simulink model "window_and_fft_test_v3"  (R2012b)
settings: Solver=ode45  StartTime=0.0  StopTime=100000  RelTol=1e-3
values from neighbouring files (symbols this model uses):
  Fs = 640e6    (= 640000000)    [filter_coefficients.m]    (also in filter_design.m; filter_design_getting_order.m)
undefined symbols (not defined in the file or in its folder): get, pfb_coeff_gen_calc, sided, Two, xlipgetpartsetting
undefined symbols (not defined in the file): A_cos, A_sin, B_cos, B_sin, C_cos, C_sin, casper_coef, D_cos, D_sin
libraries: xbsIndex_r4 x6921, casper_library_misc x45, casper_library_delays x25, dspsnks4 x17, dspspect3 x8, dspsigops x4, xps_library x2, xbsReplacements_r4 x2, casper_library_pfbs x2, simulink x1
(part 2 of 85)

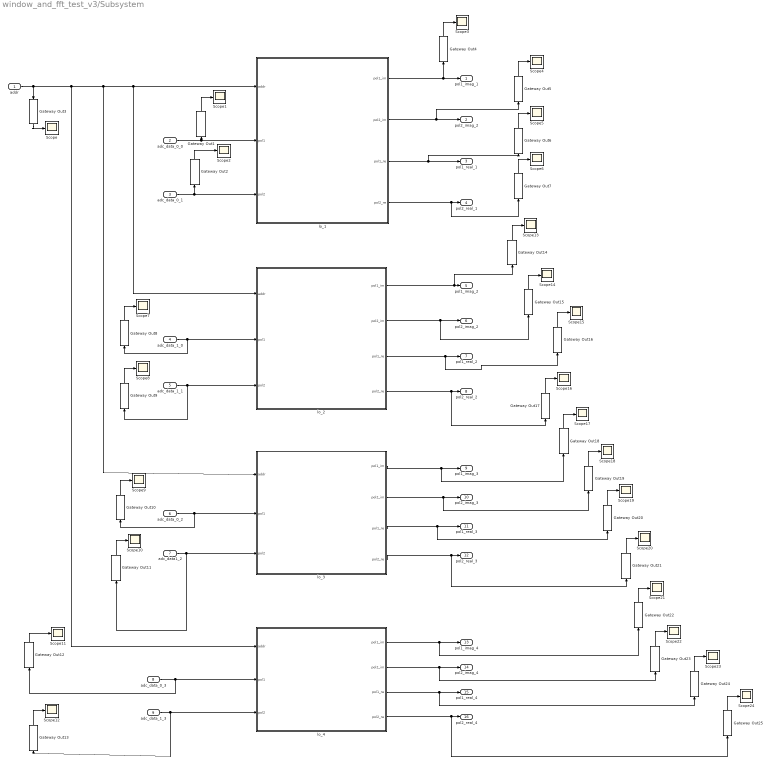
== system window_and_fft_test_v3/Subsystem ==
  addr : Inport
  adc_data_0_0 : Inport  Port=2
  adc_data_0_1 : Inport  Port=3
  adc_data_1_0 : Inport  Port=4
  adc_data_1_1 : Inport  Port=5
  adc_data_0_2 : Inport  Port=6
  adc_data1_2 : Inport  Port=7
  adc_data_0_3 : Inport  Port=8
  adc_data_1_3 : Inport  Port=9
  Gateway Out{1..25} (25 alike) : xbsIndex_r4/Gateway Out  inherit_from_input=on  hdl_port=on  timing_constraint=None  locs_specified=off  LOCs={}  UseAsDAC=off  DACChannel='1'  block_type=gatewayout
  Scope{,1..24} (25 alike) : Scope
      Scope settings: SaveName=ScopeData4
      Scope1 settings: YMin=-0.11  YMax=0.11  SaveName=ScopeData5
      Scope10 settings: YMin=-0.11  YMax=0.11  SaveName=ScopeData19
      Scope11 settings: YMin=-0.11  YMax=0.11  SaveName=ScopeData20
      Scope12 settings: YMin=-0.11  YMax=0.11  SaveName=ScopeData21
      Scope13 settings: YMin=-0.11  YMax=0.11  SaveName=ScopeData22
      Scope14 settings: YMin=-0.11  YMax=0.11  SaveName=ScopeData23
      Scope15 settings: YMin=-0.11  YMax=0.11  SaveName=ScopeData24
      Scope16 settings: YMin=-0.11  YMax=0.11  SaveName=ScopeData25
      Scope17 settings: YMin=-0.11  YMax=0.11  SaveName=ScopeData26
      Scope18 settings: YMin=-0.11  YMax=0.11  SaveName=ScopeData27
      Scope19 settings: YMin=-0.11  YMax=0.11  SaveName=ScopeData28
      Scope2 settings: YMin=-0.11  YMax=0.11  SaveName=ScopeData6
      Scope20 settings: YMin=-0.11  YMax=0.11  SaveName=ScopeData29
      Scope21 settings: YMin=-0.11  YMax=0.11  SaveName=ScopeData30
      Scope22 settings: YMin=-0.11  YMax=0.11  SaveName=ScopeData31
      Scope23 settings: YMin=-0.11  YMax=0.11  SaveName=ScopeData32
      Scope24 settings: YMin=-0.11  YMax=0.11  SaveName=ScopeData33
      Scope3 settings: YMin=-0.11  YMax=0.11  SaveName=ScopeData12
      Scope4 settings: YMin=-0.11  YMax=0.11  SaveName=ScopeData13
      Scope5 settings: YMin=-0.11  YMax=0.11  SaveName=ScopeData14
      Scope6 settings: YMin=-0.11  YMax=0.11  SaveName=ScopeData15
      Scope7 settings: YMin=-0.11  YMax=0.11  SaveName=ScopeData16
      Scope8 settings: YMin=-0.11  YMax=0.11  SaveName=ScopeData17
      Scope9 settings: YMin=-0.11  YMax=0.11  SaveName=ScopeData18
  lo_1 : Subsystem  AncestorBlock=gbt_library/complex_mix_lo
  lo_2 : Subsystem  AncestorBlock=gbt_library/complex_mix_lo
  lo_3 : Subsystem  AncestorBlock=gbt_library/complex_mix_lo
  lo_4 : Subsystem  AncestorBlock=gbt_library/complex_mix_lo
  pol1_imag_1 : Outport
  pol2_imag_2 : Outport  Port=2
  pol1_real_1 : Outport  Port=3
  pol2_real_1 : Outport  Port=4
  pol1_imag_2 : Outport  Port=5
  "pol2_imag_2 " : Outport  Port=6
  pol1_real_2 : Outport  Port=7
  pol2_real_2 : Outport  Port=8
  pol1_imag_3 : Outport  Port=9
  pol2_imag_3 : Outport  Port=10
  pol1_real_3 : Outport  Port=11
  pol2_real_3 : Outport  Port=12
  pol1_imag_4 : Outport  Port=13
  pol2_imag_4 : Outport  Port=14
  pol1_real_4 : Outport  Port=15
  pol2_real_4 : Outport  Port=16
  wires:
  lo_1/3(pol1_re) -> Gateway Out6/1, pol1_real_1/1
  lo_4/4(pol2_re) -> Gateway Out25/1, pol2_real_4/1
  adc_data_0_1/1 -> lo_1/3(pol2), Gateway Out2/1
  adc_data_1_0/1 -> lo_2/2(pol1), Gateway Out8/1
  lo_4/2(pol2_im) -> Gateway Out23/1, pol2_imag_4/1
  lo_3/4(pol2_re) -> Gateway Out21/1, pol2_real_3/1
  adc_data_1_3/1 -> lo_4/3(pol2), Gateway Out13/1
  lo_1/1(pol1_im) -> Gateway Out4/1, pol1_imag_1/1
  adc_data1_2/1 -> lo_3/3(pol2), Gateway Out11/1
  lo_2/1(pol1_im) -> Gateway Out14/1, pol1_imag_2/1
  lo_1/4(pol2_re) -> Gateway Out7/1, pol2_real_1/1
  adc_data_0_0/1 -> lo_1/2(pol1), Gateway Out1/1
  lo_1/2(pol2_im) -> Gateway Out5/1, pol2_imag_2/1
  lo_4/1(pol1_im) -> Gateway Out22/1, pol1_imag_4/1
  adc_data_0_2/1 -> Gateway Out10/1, lo_3/2(pol1)
  adc_data_1_1/1 -> lo_2/3(pol2), Gateway Out9/1
  lo_2/4(pol2_re) -> Gateway Out17/1, pol2_real_2/1
  addr/1 -> Gateway Out3/1, lo_4/1(addr), lo_2/1(addr), lo_1/1(addr), lo_3/1(addr)
  lo_3/1(pol1_im) -> Gateway Out18/1, pol1_imag_3/1
  lo_2/2(pol2_im) -> Gateway Out15/1, "pol2_imag_2 "/1
  Gateway Out3/1 -> Scope/1
  Gateway Out1/1 -> Scope1/1
  Gateway Out2/1 -> Scope2/1
  Gateway Out4/1 -> Scope3/1
  Gateway Out5/1 -> Scope4/1
  Gateway Out6/1 -> Scope5/1
  Gateway Out7/1 -> Scope6/1
  Gateway Out8/1 -> Scope7/1
  Gateway Out9/1 -> Scope8/1
  Gateway Out10/1 -> Scope9/1
  Gateway Out11/1 -> Scope10/1
  Gateway Out12/1 -> Scope11/1
  adc_data_0_3/1 -> Gateway Out12/1, lo_4/2(pol1)
  Gateway Out13/1 -> Scope12/1
  Gateway Out14/1 -> Scope13/1
  Gateway Out15/1 -> Scope14/1
  Gateway Out16/1 -> Scope15/1
  lo_2/3(pol1_re) -> Gateway Out16/1, pol1_real_2/1
  Gateway Out17/1 -> Scope16/1
  Gateway Out18/1 -> Scope17/1
  Gateway Out19/1 -> Scope18/1
  lo_3/2(pol2_im) -> Gateway Out19/1, pol2_imag_3/1
  Gateway Out20/1 -> Scope19/1
  lo_3/3(pol1_re) -> Gateway Out20/1, pol1_real_3/1
  Gateway Out21/1 -> Scope20/1
  Gateway Out22/1 -> Scope21/1
  Gateway Out23/1 -> Scope22/1
  Gateway Out24/1 -> Scope23/1
  lo_4/3(pol1_re) -> Gateway Out24/1, pol1_real_4/1
  Gateway Out25/1 -> Scope24/1

== system window_and_fft_test_v3/bypass_pfb ==
  sim_1 : Inport
  io_delay : xbsIndex_r4/Delay  rst=off  infoeditControl=Selection of Reset will increase slice count due to use of real FFs and instead of SRLs  en=off  latency=0  dbl_ovrd=off  reg_retiming=on  block_type=delay
  reint1 : xbsIndex_r4/Reinterpret  force_arith_type=on  arith_type=Unsigned  force_bin_pt=on  bin_pt=0  block_type=reinterpret
  slice_reg : xbsIndex_r4/Slice  nbits=11  boolean_output=off  mode=Lower Bit Location + Width  bit1=0  base1=MSB of Input  bit0=0  base0=LSB of Input  dbl_ovrd=off  block_type=slice
  window_and_fft_test_v3_bypass_pfb_user_data_out : xbsIndex_r4/Gateway In  gui_display_data_type=Fixed-point  arith_type=Unsigned  n_bits=32  bin_pt=0  preci_type=Single  exp_width=8  frac_width=24  quantization="Round  (unbiased: +/- Inf)"  overflow=Saturate  period=1  dbl_ovrd=off  timing_constraint=None  locs_specified=off  LOCs={}  UseAsADC=off  ADCChannel='1'  inherit_from_input=off  hdl_port=on  block_type=gatewayin
  in_reg : Outport
  wires:
  window_and_fft_test_v3_bypass_pfb_user_data_out/1 -> io_delay/1
  sim_1/1 -> window_and_fft_test_v3_bypass_pfb_user_data_out/1
  io_delay/1 -> slice_reg/1
  slice_reg/1 -> reint1/1
  reint1/1 -> in_reg/1

== system window_and_fft_test_v3/coarse_fft_shift_mask1 ==
  sim_1 : Inport
  io_delay : xbsIndex_r4/Delay  rst=off  infoeditControl=Selection of Reset will increase slice count due to use of real FFs and instead of SRLs  en=off  latency=0  dbl_ovrd=off  reg_retiming=on  block_type=delay
  reint1 : xbsIndex_r4/Reinterpret  force_arith_type=on  arith_type=Unsigned  force_bin_pt=on  bin_pt=0  block_type=reinterpret
  slice_reg : xbsIndex_r4/Slice  nbits=11  boolean_output=off  mode=Lower Bit Location + Width  bit1=0  base1=MSB of Input  bit0=0  base0=LSB of Input  dbl_ovrd=off  block_type=slice
  window_and_fft_test_v3_coarse_fft_shift_mask1_user_data_out : xbsIndex_r4/Gateway In  gui_display_data_type=Fixed-point  arith_type=Unsigned  n_bits=32  bin_pt=0  preci_type=Single  exp_width=8  frac_width=24  quantization="Round  (unbiased: +/- Inf)"  overflow=Saturate  period=1  dbl_ovrd=off  timing_constraint=None  locs_specified=off  LOCs={}  UseAsADC=off  ADCChannel='1'  inherit_from_input=off  hdl_port=on  block_type=gatewayin
  in_reg : Outport
  wires:
  window_and_fft_test_v3_coarse_fft_shift_mask1_user_data_out/1 -> io_delay/1
  sim_1/1 -> window_and_fft_test_v3_coarse_fft_shift_mask1_user_data_out/1
  io_delay/1 -> slice_reg/1
  slice_reg/1 -> reint1/1
  reint1/1 -> in_reg/1

== system window_and_fft_test_v3/convert_of10 ==
  din : Inport
  convert : xbsIndex_r4/Convert  gui_display_data_type=Fixed-point  arith_type="Signed  (2's comp)"  n_bits=bit_width_o  bin_pt=binary_point_o  float_type=Single  exp_bits=8  fraction_bits=24  quantization=Truncate  overflow=Wrap  en=off  latency=latency  dbl_ovrd=off  pipeline=on  block_type=convert
  never : xbsIndex_r4/Constant  const=0  gui_display_data_type=Fixed-point  arith_type=Boolean  n_bits=16  bin_pt=14  preci_type=Single  exp_width=8  frac_width=24  explicit_period=on  period=1  equ=P=C  opselect=C  inp2=PCIN>>17  opr=+  inp1=P  carry=CIN  dbl_ovrd=off  block_type=constant
  dout : Outport
  of : Outport  Port=2
  wires:
  never/1 -> of/1
  convert/1 -> dout/1
  din/1 -> convert/1

== system window_and_fft_test_v3/convert_of11 ==
  din : Inport
  convert : xbsIndex_r4/Convert  gui_display_data_type=Fixed-point  arith_type="Signed  (2's comp)"  n_bits=bit_width_o  bin_pt=binary_point_o  float_type=Single  exp_bits=8  fraction_bits=24  quantization=Truncate  overflow=Wrap  en=off  latency=latency  dbl_ovrd=off  pipeline=on  block_type=convert
  never : xbsIndex_r4/Constant  const=0  gui_display_data_type=Fixed-point  arith_type=Boolean  n_bits=16  bin_pt=14  preci_type=Single  exp_width=8  frac_width=24  explicit_period=on  period=1  equ=P=C  opselect=C  inp2=PCIN>>17  opr=+  inp1=P  carry=CIN  dbl_ovrd=off  block_type=constant
  dout : Outport
  of : Outport  Port=2
  wires:
  din/1 -> convert/1
  convert/1 -> dout/1
  never/1 -> of/1

== system window_and_fft_test_v3/convert_of8 ==
  din : Inport
  convert : xbsIndex_r4/Convert  gui_display_data_type=Fixed-point  arith_type="Signed  (2's comp)"  n_bits=bit_width_o  bin_pt=binary_point_o  float_type=Single  exp_bits=8  fraction_bits=24  quantization=Truncate  overflow=Wrap  en=off  latency=latency  dbl_ovrd=off  pipeline=on  block_type=convert
  never : xbsIndex_r4/Constant  const=0  gui_display_data_type=Fixed-point  arith_type=Boolean  n_bits=16  bin_pt=14  preci_type=Single  exp_width=8  frac_width=24  explicit_period=on  period=1  equ=P=C  opselect=C  inp2=PCIN>>17  opr=+  inp1=P  carry=CIN  dbl_ovrd=off  block_type=constant
  dout : Outport
  of : Outport  Port=2
  wires:
  din/1 -> convert/1
  convert/1 -> dout/1
  never/1 -> of/1

== system window_and_fft_test_v3/convert_of9 ==
  din : Inport
  convert : xbsIndex_r4/Convert  gui_display_data_type=Fixed-point  arith_type="Signed  (2's comp)"  n_bits=bit_width_o  bin_pt=binary_point_o  float_type=Single  exp_bits=8  fraction_bits=24  quantization=Truncate  overflow=Wrap  en=off  latency=latency  dbl_ovrd=off  pipeline=on  block_type=convert
  never : xbsIndex_r4/Constant  const=0  gui_display_data_type=Fixed-point  arith_type=Boolean  n_bits=16  bin_pt=14  preci_type=Single  exp_width=8  frac_width=24  explicit_period=on  period=1  equ=P=C  opselect=C  inp2=PCIN>>17  opr=+  inp1=P  carry=CIN  dbl_ovrd=off  block_type=constant
  dout : Outport
  of : Outport  Port=2
  wires:
  din/1 -> convert/1
  convert/1 -> dout/1
  never/1 -> of/1

== system window_and_fft_test_v3/dec_fir ==
  sync_in : Inport
  real1 : Inport  Port=2
  imag1 : Inport  Port=3
  real2 : Inport  Port=4
  imag2 : Inport  Port=5
  real3 : Inport  Port=6
  imag3 : Inport  Port=7
  real4 : Inport  Port=8
  imag4 : Inport  Port=9
  convert1 : xbsIndex_r4/Convert  gui_display_data_type=Fixed-point  arith_type="Signed  (2's comp)"  n_bits=16  bin_pt=15  float_type=Single  exp_bits=8  fraction_bits=24  quantization="Round  (unbiased: +/- Inf)"  overflow=Wrap  en=off  latency=2  dbl_ovrd=off  pipeline=off  block_type=convert
  convert2 : xbsIndex_r4/Convert  gui_display_data_type=Fixed-point  arith_type="Signed  (2's comp)"  n_bits=16  bin_pt=15  float_type=Single  exp_bits=8  fraction_bits=24  quantization="Round  (unbiased: +/- Inf)"  overflow=Wrap  en=off  latency=2  dbl_ovrd=off  pipeline=off  block_type=convert
  delay : xbsIndex_r4/Delay  rst=off  infoeditControl=Selection of Reset will increase slice count due to use of real FFs and instead of SRLs  en=off  latency=7  dbl_ovrd=off  reg_retiming=off  block_type=delay
  fir_dbl_col1 : Subsystem  AncestorBlock=casper_library_downconverter/fir_dbl_col  mask(fir_dbl_col){n_inputs=4, coeff=[0.037109    0.023207    0.012354   0.0056253], add_latency=1, mult_latency=2, coeff_bit_width=25, coeff_bin_pt=24, first_stage_hdl=on, adder_imp=DSP48}
      mask prompts: n_inputs "Inputs"; coeff "Coefficients"; add_latency "Add latency"; mult_latency "Mult Latency"; coeff_bit_width "Coefficient bit width"; coeff_bin_pt "Coefficient binary point"; first_stage_hdl "Implement first stage of adder trees on output as behavioural HDL"; adder_imp "Adder implementation"
      mask init:
      | fir_dbl_col_init(gcb, ...
      |     'n_inputs', n_inputs, ...
      |     'coeff', coeff, ...
      |     'mult_latency', mult_latency, ...
      |     'add_latency', add_latency, ...
      |     'coeff_bit_width', coeff_bit_width, ...
      |     'coeff_bin_pt', coeff_bin_pt,  ...
      |     'first_stage_hdl', first_stage_hdl, ...
      |     'adder_imp', adder_imp);
      mask Help: eval('xlWeb(''http://casper.berkeley.edu/wiki/Fir_dbl_col'')')
      mask TypeOptions adder_imp: Behavioral | Fabric | DSP48
  fir_dbl_col2 : Subsystem  AncestorBlock=casper_library_downconverter/fir_dbl_col  mask(fir_dbl_col){n_inputs=4, coeff=[0.08556    0.079092    0.067391    0.052572], add_latency=1, mult_latency=2, coeff_bit_width=25, coeff_bin_pt=24, first_stage_hdl=on, adder_imp=DSP48}
      mask prompts: n_inputs "Inputs"; coeff "Coefficients"; add_latency "Add latency"; mult_latency "Mult Latency"; coeff_bit_width "Coefficient bit width"; coeff_bin_pt "Coefficient binary point"; first_stage_hdl "Implement first stage of adder trees on output as behavioural HDL"; adder_imp "Adder implementation"
      mask init: same as window_and_fft_test_v3/dec_fir/fir_dbl_col1
      mask Help: eval('xlWeb(''http://casper.berkeley.edu/wiki/Fir_dbl_col'')')
      mask TypeOptions adder_imp: Behavioral | Fabric | DSP48
  imag_sum : Subsystem  AncestorBlock=casper_library_misc/adder_tree  mask(adder_tree){n_inputs=2, latency=1, adder_imp=DSP48, first_stage_hdl=off}
      mask prompts: n_inputs "Number of Inputs"; latency "Add Latency"; adder_imp "Adder implementation"; first_stage_hdl "Use behavioural HDL for first stage of adders"
      mask help:
      | Sums all inputs using a tree of adds and delays.
      |
      | Number of inputs: The number of inputs to the block to be summed
      | Add latency: The number of clock cycles to perform one addition (affects timing)..
      | Adder implementation: choice of fabric or DSP48E core, or behavioral HDL
      | Use behavioural HDL for first stage of adders: Causes the first stage of adders to be absorbed into DSP blocks if multipliers precede them (Virtex 5). Overrides Adder implementation
      mask init:
      | adder_tree_init(gcb, ...
      |     'n_inputs', n_inputs, ...
      |     'latency', latency, ...
      |     'adder_imp', adder_imp, ...
      |     'first_stage_hdl', first_stage_hdl);
      settings: AttributesFormatString=latency 1
      mask Help: eval('xlWeb(''http://casper.berkeley.edu/wiki/Adder_tree'')')
      mask TypeOptions adder_imp: Behavioral | Fabric | DSP48
  real_sum : Subsystem  AncestorBlock=casper_library_misc/adder_tree  mask(adder_tree){n_inputs=2, latency=1, adder_imp=DSP48, first_stage_hdl=off}
      mask prompts: n_inputs "Number of Inputs"; latency "Add Latency"; adder_imp "Adder implementation"; first_stage_hdl "Use behavioural HDL for first stage of adders"
      mask help:
      | Sums all inputs using a tree of adds and delays.
      |
      | Number of inputs: The number of inputs to the block to be summed
      | Add latency: The number of clock cycles to perform one addition (affects timing)..
      | Adder implementation: choice of fabric or DSP48E core, or behavioral HDL
      | Use behavioural HDL for first stage of adders: Causes the first stage of adders to be absorbed into DSP blocks if multipliers precede them (Virtex 5). Overrides Adder implementation
      mask init:
      | adder_tree_init(gcb, ...
      |     'n_inputs', n_inputs, ...
      |     'latency', latency, ...
      |     'adder_imp', adder_imp, ...
      |     'first_stage_hdl', first_stage_hdl);
      settings: AttributesFormatString=latency 1
      mask Help: eval('xlWeb(''http://casper.berkeley.edu/wiki/Adder_tree'')')
      mask TypeOptions adder_imp: Behavioral | Fabric | DSP48
  ri_to_c : casper_library_misc/ri_to_c
  shift1 : xbsIndex_r4/Shift  shift_dir=Left  shift_bits=1  en=off  latency=0  precision=Full  arith_type="Signed  (2's comp)"  n_bits=16  bin_pt=14  quantization=Truncate  overflow=Wrap  dbl_ovrd=off  block_type=shift
  shift2 : xbsIndex_r4/Shift  shift_dir=Left  shift_bits=1  en=off  latency=0  precision=Full  arith_type="Signed  (2's comp)"  n_bits=16  bin_pt=14  quantization=Truncate  overflow=Wrap  dbl_ovrd=off  block_type=shift
  sync_out : Outport
  dout : Outport  Port=2
  wires:
  real1/1 -> fir_dbl_col1/1(real1)
  imag1/1 -> fir_dbl_col1/2(imag1)
  real2/1 -> fir_dbl_col1/3(real2)
  imag2/1 -> fir_dbl_col1/4(imag2)
  real3/1 -> fir_dbl_col1/5(real3)
  imag3/1 -> fir_dbl_col1/6(imag3)
  real4/1 -> fir_dbl_col1/7(real4)
  imag4/1 -> fir_dbl_col1/8(imag4)
  fir_dbl_col1/17(real_sum) -> real_sum/2(din1)
  fir_dbl_col1/18(imag_sum) -> imag_sum/2(din1)
  fir_dbl_col1/1(real_out1) -> fir_dbl_col2/1(real1)
  fir_dbl_col1/2(imag_out1) -> fir_dbl_col2/2(imag1)
  fir_dbl_col1/3(real_out2) -> fir_dbl_col2/3(real2)
  fir_dbl_col1/4(imag_out2) -> fir_dbl_col2/4(imag2)
  fir_dbl_col1/5(real_out3) -> fir_dbl_col2/5(real3)
  fir_dbl_col1/6(imag_out3) -> fir_dbl_col2/6(imag3)
  fir_dbl_col1/7(real_out4) -> fir_dbl_col2/7(real4)
  fir_dbl_col1/8(imag_out4) -> fir_dbl_col2/8(imag4)
  fir_dbl_col2/17(real_sum) -> real_sum/3(din2)
  fir_dbl_col2/18(imag_sum) -> imag_sum/3(din2)
  real_sum/2(dout) -> shift1/1
  imag_sum/2(dout) -> shift2/1
  shift1/1 -> convert1/1
  shift2/1 -> convert2/1
  convert1/1 -> ri_to_c/1
  convert2/1 -> ri_to_c/2
  ri_to_c/1 -> dout/1
  sync_in/1 -> delay/1
  delay/1 -> real_sum/1(sync), imag_sum/1(sync)
  real_sum/1(sync_out) -> sync_out/1
  fir_dbl_col2/9(real_back_out1) -> fir_dbl_col1/9(real_back1)
  fir_dbl_col2/10(imag_back_out1) -> fir_dbl_col1/10(imag_back1)
  fir_dbl_col2/11(real_back_out2) -> fir_dbl_col1/11(real_back2)
  fir_dbl_col2/12(imag_back_out2) -> fir_dbl_col1/12(imag_back2)
  fir_dbl_col2/13(real_back_out3) -> fir_dbl_col1/13(real_back3)
  fir_dbl_col2/14(imag_back_out3) -> fir_dbl_col1/14(imag_back3)
  fir_dbl_col2/15(real_back_out4) -> fir_dbl_col1/15(real_back4)
  fir_dbl_col2/16(imag_back_out4) -> fir_dbl_col1/16(imag_back4)
  fir_dbl_col2/1(real_out1) -> fir_dbl_col2/9(real_back1)
  fir_dbl_col2/2(imag_out1) -> fir_dbl_col2/10(imag_back1)
  fir_dbl_col2/3(real_out2) -> fir_dbl_col2/11(real_back2)
  fir_dbl_col2/4(imag_out2) -> fir_dbl_col2/12(imag_back2)
  fir_dbl_col2/5(real_out3) -> fir_dbl_col2/13(real_back3)
  fir_dbl_col2/6(imag_out3) -> fir_dbl_col2/14(imag_back3)
  fir_dbl_col2/7(real_out4) -> fir_dbl_col2/15(real_back4)
  fir_dbl_col2/8(imag_out4) -> fir_dbl_col2/16(imag_back4)

== system window_and_fft_test_v3/dec_fir1 ==
  sync_in : Inport
  real1 : Inport  Port=2
  imag1 : Inport  Port=3
  real2 : Inport  Port=4
  imag2 : Inport  Port=5
  real3 : Inport  Port=6
  imag3 : Inport  Port=7
  real4 : Inport  Port=8
  imag4 : Inport  Port=9
  convert1 : xbsIndex_r4/Convert  gui_display_data_type=Fixed-point  arith_type="Signed  (2's comp)"  n_bits=16  bin_pt=15  float_type=Single  exp_bits=8  fraction_bits=24  quantization="Round  (unbiased: +/- Inf)"  overflow=Wrap  en=off  latency=2  dbl_ovrd=off  pipeline=off  block_type=convert
  convert2 : xbsIndex_r4/Convert  gui_display_data_type=Fixed-point  arith_type="Signed  (2's comp)"  n_bits=16  bin_pt=15  float_type=Single  exp_bits=8  fraction_bits=24  quantization="Round  (unbiased: +/- Inf)"  overflow=Wrap  en=off  latency=2  dbl_ovrd=off  pipeline=off  block_type=convert
  delay : xbsIndex_r4/Delay  rst=off  infoeditControl=Selection of Reset will increase slice count due to use of real FFs and instead of SRLs  en=off  latency=7  dbl_ovrd=off  reg_retiming=off  block_type=delay
  fir_dbl_col1 : Subsystem  AncestorBlock=casper_library_downconverter/fir_dbl_col  mask(fir_dbl_col){n_inputs=4, coeff=[0.037109    0.023207    0.012354   0.0056253], add_latency=1, mult_latency=2, coeff_bit_width=25, coeff_bin_pt=24, first_stage_hdl=on, adder_imp=DSP48}
      mask prompts: n_inputs "Inputs"; coeff "Coefficients"; add_latency "Add latency"; mult_latency "Mult Latency"; coeff_bit_width "Coefficient bit width"; coeff_bin_pt "Coefficient binary point"; first_stage_hdl "Implement first stage of adder trees on output as behavioural HDL"; adder_imp "Adder implementation"
      mask init: same as window_and_fft_test_v3/dec_fir/fir_dbl_col1
      mask Help: eval('xlWeb(''http://casper.berkeley.edu/wiki/Fir_dbl_col'')')
      mask TypeOptions adder_imp: Behavioral | Fabric | DSP48
  fir_dbl_col2 : Subsystem  AncestorBlock=casper_library_downconverter/fir_dbl_col  mask(fir_dbl_col){n_inputs=4, coeff=[0.08556    0.079092    0.067391    0.052572], add_latency=1, mult_latency=2, coeff_bit_width=25, coeff_bin_pt=24, first_stage_hdl=on, adder_imp=DSP48}
      mask prompts: n_inputs "Inputs"; coeff "Coefficients"; add_latency "Add latency"; mult_latency "Mult Latency"; coeff_bit_width "Coefficient bit width"; coeff_bin_pt "Coefficient binary point"; first_stage_hdl "Implement first stage of adder trees on output as behavioural HDL"; adder_imp "Adder implementation"
      mask init: same as window_and_fft_test_v3/dec_fir/fir_dbl_col1
      mask Help: eval('xlWeb(''http://casper.berkeley.edu/wiki/Fir_dbl_col'')')
      mask TypeOptions adder_imp: Behavioral | Fabric | DSP48
  imag_sum : Subsystem  AncestorBlock=casper_library_misc/adder_tree  mask(adder_tree){n_inputs=2, latency=1, adder_imp=DSP48, first_stage_hdl=off}
      mask prompts: n_inputs "Number of Inputs"; latency "Add Latency"; adder_imp "Adder implementation"; first_stage_hdl "Use behavioural HDL for first stage of adders"
      mask help:
      | Sums all inputs using a tree of adds and delays.
      |
      | Number of inputs: The number of inputs to the block to be summed
      | Add latency: The number of clock cycles to perform one addition (affects timing)..
      | Adder implementation: choice of fabric or DSP48E core, or behavioral HDL
      | Use behavioural HDL for first stage of adders: Causes the first stage of adders to be absorbed into DSP blocks if multipliers precede them (Virtex 5). Overrides Adder implementation
      mask init:
      | adder_tree_init(gcb, ...
      |     'n_inputs', n_inputs, ...
      |     'latency', latency, ...
      |     'adder_imp', adder_imp, ...
      |     'first_stage_hdl', first_stage_hdl);
      settings: AttributesFormatString=latency 1
      mask Help: eval('xlWeb(''http://casper.berkeley.edu/wiki/Adder_tree'')')
      mask TypeOptions adder_imp: Behavioral | Fabric | DSP48
  real_sum : Subsystem  AncestorBlock=casper_library_misc/adder_tree  mask(adder_tree){n_inputs=2, latency=1, adder_imp=DSP48, first_stage_hdl=off}
      mask prompts: n_inputs "Number of Inputs"; latency "Add Latency"; adder_imp "Adder implementation"; first_stage_hdl "Use behavioural HDL for first stage of adders"
      mask help:
      | Sums all inputs using a tree of adds and delays.
      |
      | Number of inputs: The number of inputs to the block to be summed
      | Add latency: The number of clock cycles to perform one addition (affects timing)..
      | Adder implementation: choice of fabric or DSP48E core, or behavioral HDL
      | Use behavioural HDL for first stage of adders: Causes the first stage of adders to be absorbed into DSP blocks if multipliers precede them (Virtex 5). Overrides Adder implementation
      mask init:
      | adder_tree_init(gcb, ...
      |     'n_inputs', n_inputs, ...
      |     'latency', latency, ...
      |     'adder_imp', adder_imp, ...
      |     'first_stage_hdl', first_stage_hdl);
      settings: AttributesFormatString=latency 1
      mask Help: eval('xlWeb(''http://casper.berkeley.edu/wiki/Adder_tree'')')
      mask TypeOptions adder_imp: Behavioral | Fabric | DSP48
  ri_to_c : casper_library_misc/ri_to_c
  shift1 : xbsIndex_r4/Shift  shift_dir=Left  shift_bits=1  en=off  latency=0  precision=Full  arith_type="Signed  (2's comp)"  n_bits=16  bin_pt=14  quantization=Truncate  overflow=Wrap  dbl_ovrd=off  block_type=shift
  shift2 : xbsIndex_r4/Shift  shift_dir=Left  shift_bits=1  en=off  latency=0  precision=Full  arith_type="Signed  (2's comp)"  n_bits=16  bin_pt=14  quantization=Truncate  overflow=Wrap  dbl_ovrd=off  block_type=shift
  sync_out : Outport
  dout : Outport  Port=2
  wires:
  real1/1 -> fir_dbl_col1/1(real1)
  imag1/1 -> fir_dbl_col1/2(imag1)
  real2/1 -> fir_dbl_col1/3(real2)
  imag2/1 -> fir_dbl_col1/4(imag2)
  real3/1 -> fir_dbl_col1/5(real3)
  imag3/1 -> fir_dbl_col1/6(imag3)
  real4/1 -> fir_dbl_col1/7(real4)
  imag4/1 -> fir_dbl_col1/8(imag4)
  fir_dbl_col1/17(real_sum) -> real_sum/2(din1)
  fir_dbl_col1/18(imag_sum) -> imag_sum/2(din1)
  fir_dbl_col1/1(real_out1) -> fir_dbl_col2/1(real1)
  fir_dbl_col1/2(imag_out1) -> fir_dbl_col2/2(imag1)
  fir_dbl_col1/3(real_out2) -> fir_dbl_col2/3(real2)
  fir_dbl_col1/4(imag_out2) -> fir_dbl_col2/4(imag2)
  fir_dbl_col1/5(real_out3) -> fir_dbl_col2/5(real3)
  fir_dbl_col1/6(imag_out3) -> fir_dbl_col2/6(imag3)
  fir_dbl_col1/7(real_out4) -> fir_dbl_col2/7(real4)
  fir_dbl_col1/8(imag_out4) -> fir_dbl_col2/8(imag4)
  fir_dbl_col2/17(real_sum) -> real_sum/3(din2)
  fir_dbl_col2/18(imag_sum) -> imag_sum/3(din2)
  real_sum/2(dout) -> shift1/1
  imag_sum/2(dout) -> shift2/1
  shift1/1 -> convert1/1
  shift2/1 -> convert2/1
  convert1/1 -> ri_to_c/1
  convert2/1 -> ri_to_c/2
  ri_to_c/1 -> dout/1
  sync_in/1 -> delay/1
  delay/1 -> real_sum/1(sync), imag_sum/1(sync)
  real_sum/1(sync_out) -> sync_out/1
  fir_dbl_col2/9(real_back_out1) -> fir_dbl_col1/9(real_back1)
  fir_dbl_col2/10(imag_back_out1) -> fir_dbl_col1/10(imag_back1)
  fir_dbl_col2/11(real_back_out2) -> fir_dbl_col1/11(real_back2)
  fir_dbl_col2/12(imag_back_out2) -> fir_dbl_col1/12(imag_back2)
  fir_dbl_col2/13(real_back_out3) -> fir_dbl_col1/13(real_back3)
  fir_dbl_col2/14(imag_back_out3) -> fir_dbl_col1/14(imag_back3)
  fir_dbl_col2/15(real_back_out4) -> fir_dbl_col1/15(real_back4)
  fir_dbl_col2/16(imag_back_out4) -> fir_dbl_col1/16(imag_back4)
  fir_dbl_col2/1(real_out1) -> fir_dbl_col2/9(real_back1)
  fir_dbl_col2/2(imag_out1) -> fir_dbl_col2/10(imag_back1)
  fir_dbl_col2/3(real_out2) -> fir_dbl_col2/11(real_back2)
  fir_dbl_col2/4(imag_out2) -> fir_dbl_col2/12(imag_back2)
  fir_dbl_col2/5(real_out3) -> fir_dbl_col2/13(real_back3)
  fir_dbl_col2/6(imag_out3) -> fir_dbl_col2/14(imag_back3)
  fir_dbl_col2/7(real_out4) -> fir_dbl_col2/15(real_back4)
  fir_dbl_col2/8(imag_out4) -> fir_dbl_col2/16(imag_back4)

== system window_and_fft_test_v3/even_window1 ==
  addr : Inport
  data_in : Inport  Port=2
  we : Inport  Port=3
  calc_add : Subsystem  mask{data_width=64, addr_width=10, sample_rate=sample_rate}
      mask prompts: data_width "data width"; addr_width "address width"; sample_rate "sample rate"
  convert_addr : xbsIndex_r4/Convert  gui_display_data_type=Fixed-point  arith_type=Unsigned  n_bits=addr_width  bin_pt=0  float_type=Single  exp_bits=8  fraction_bits=24  quantization=Truncate  overflow=Wrap  en=off  latency=0  dbl_ovrd=off  pipeline=off  block_type=convert
      settings: xl_area=[0, 0, 0, 0, 0, 0, 0]
  convert_din1 : xbsIndex_r4/Convert  gui_display_data_type=Fixed-point  arith_type=Unsigned  n_bits=64  bin_pt=0  float_type=Single  exp_bits=8  fraction_bits=24  quantization=Truncate  overflow=Wrap  en=off  latency=0  dbl_ovrd=off  pipeline=off  block_type=convert
      settings: xl_area=[0, 0, 0, 0, 0, 0, 0]
  convert_we : xbsIndex_r4/Convert  gui_display_data_type=Fixed-point  arith_type=Unsigned  n_bits=1  bin_pt=0  float_type=Single  exp_bits=8  fraction_bits=24  quantization=Truncate  overflow=Wrap  en=off  latency=0  dbl_ovrd=off  pipeline=off  block_type=convert
      settings: xl_area=[0, 0, 0, 0, 0, 0, 0]
  mem : Subsystem
  munge_in : Subsystem  AncestorBlock=casper_library_flow_control/munge  mask(munge){divisions=2, div_size=[32 32], order=[1  0], arith_type_out=Unsigned, bin_pt_out=0}
      mask prompts: divisions "Number of divisions"; div_size "Division size (bits)"; order "Division packing order"; arith_type_out "Output arithmetic type"; bin_pt_out "Output binary point"
      mask help: Splits an input bus into the specified number of divisions and then recombines them in the order specified (most significant division = 0,least = number divisions-1)
      mask init:
      | munge_init(gcb, ...
      |     'divisions', divisions, ...
      |     'div_size', div_size, ...
      |     'order', order, ...
      |     'arith_type_out', arith_type_out, ...
      |     'bin_pt_out', bin_pt_out);
      settings: AttributesFormatString=|
      | split:[32 32]
      | join:[1 0]
      | Unsigned [64,0]
      mask TypeOptions arith_type_out: Unsigned | Signed  (2's comp) | Floating-point
  munge_out : Subsystem  AncestorBlock=casper_library_flow_control/munge  mask(munge){divisions=2, div_size=[32 32], order=[1  0], arith_type_out=Unsigned, bin_pt_out=0}
      mask prompts: divisions "Number of divisions"; div_size "Division size (bits)"; order "Division packing order"; arith_type_out "Output arithmetic type"; bin_pt_out "Output binary point"
      mask help: Splits an input bus into the specified number of divisions and then recombines them in the order specified (most significant division = 0,least = number divisions-1)
      mask init:
      | munge_init(gcb, ...
      |     'divisions', divisions, ...
      |     'div_size', div_size, ...
      |     'order', order, ...
      |     'arith_type_out', arith_type_out, ...
      |     'bin_pt_out', bin_pt_out);
      settings: AttributesFormatString=|
      | split:[32 32]
      | join:[1 0]
      | Unsigned [64,0]
      mask TypeOptions arith_type_out: Unsigned | Signed  (2's comp) | Floating-point
  window_and_fft_test_v3_even_window1_addr : xbsIndex_r4/Gateway Out  inherit_from_input=off  hdl_port=on  timing_constraint=None  locs_specified=off  LOCs={'A5','B9','A9','C1','A3','G6','E9','A6','A7','A8','B8','B1','B3','D9','B5','B4','B6','C2'}  UseAsDAC=off  DACChannel='1'  block_type=gatewayout
      settings: infoedit="Gateway out block.  Converts Xilinx fixed point inputs into ouputs of type Simulink integer, double, or fixed point.<P><P>Hardware notes:  In hardware these blocks become top level output ports or are discarded, depending on how they are configured."  xl_area=[0, 0, 0, 0, 0, 0, 0]  sginterface={'Nallatech'=>{'xdspkit'=>{'non_memory_mapped_port'=>'uprev_Shared_BRAM_addr'}},'Xilinx'=>{'jtaghwcosim'=>{'non_memory_mapped_port'=>'uprev_Shared_BRAM_addr'},'xdspkit'=>{'non_memory_mapped_port'=>'uprev_Shared_BRAM_addr'}}}
  window_and_fft_test_v3_even_window1_data_in : xbsIndex_r4/Gateway Out  inherit_from_input=off  hdl_port=on  timing_constraint=None  locs_specified=off  LOCs={'B21','B22','A22','B23','B19','C19','A20','A21','A23','B24','A24','A25','E18','D18','C18','B18'}  UseAsDAC=off  DACChannel='1'  block_type=gatewayout
      settings: infoedit="Gateway out block.  Converts Xilinx fixed point inputs into ouputs of type Simulink integer, double, or fixed point.<P><P>Hardware notes:  In hardware these blocks become top level output ports or are discarded, depending on how they are configured."  xl_area=[0, 0, 0, 0, 0, 0, 0]  sginterface={'Nallatech'=>{'xdspkit'=>{'non_memory_mapped_port'=>'uprev_Shared_BRAM_data_in'}},'Xilinx'=>{'jtaghwcosim'=>{'non_memory_mapped_port'=>'uprev_Shared_BRAM_data_in'},'xdspkit'=>{'non_memory_mapped_port'=>'uprev_Shared_BRAM_data_in'}}}
  window_and_fft_test_v3_even_window1_data_out : xbsIndex_r4/Gateway In  gui_display_data_type=Fixed-point  arith_type=Unsigned  n_bits=64  bin_pt=0  preci_type=Single  exp_width=8  frac_width=24  quantization=Truncate  overflow=Wrap  period=sample_rate  dbl_ovrd=off  timing_constraint=None  locs_specified=off  LOCs={}  UseAsADC=off  ADCChannel='1'  inherit_from_input=off  hdl_port=on  block_type=gatewayin
      settings: xl_area=[0, 0, 0, 0, 0, 0, 0]
  window_and_fft_test_v3_even_window1_we : xbsIndex_r4/Gateway Out  inherit_from_input=off  hdl_port=on  timing_constraint=None  locs_specified=off  LOCs={'A14'}  UseAsDAC=off  DACChannel='1'  block_type=gatewayout
      settings: infoedit="Gateway out block.  Converts Xilinx fixed point inputs into ouputs of type Simulink integer, double, or fixed point.<P><P>Hardware notes:  In hardware these blocks become top level output ports or are discarded, depending on how they are configured."  xl_area=[0, 0, 0, 0, 0, 0, 0]
  data_out : Outport
  wires:
  convert_addr/1 -> window_and_fft_test_v3_even_window1_addr/1
  convert_din1/1 -> window_and_fft_test_v3_even_window1_data_in/1
  data_in/1 -> munge_in/1(din)
  calc_add/1(out) -> convert_addr/1
  window_and_fft_test_v3_even_window1_we/1 -> mem/3(In3)
  window_and_fft_test_v3_even_window1_data_in/1 -> mem/2(In2)
  window_and_fft_test_v3_even_window1_addr/1 -> mem/1(In1)
  convert_we/1 -> window_and_fft_test_v3_even_window1_we/1
  window_and_fft_test_v3_even_window1_data_out/1 -> munge_out/1(din)
  mem/1(Out1) -> window_and_fft_test_v3_even_window1_data_out/1
  addr/1 -> calc_add/1(in)
  we/1 -> convert_we/1
  munge_out/1(dout) -> data_out/1
  munge_in/1(dout) -> convert_din1/1
